simulink model "lift_stateflow"  (R2020b)
settings: Solver=VariableStepAuto  StartTime=0.0  StopTime=10.0  RelTol=1e-3
undefined symbols (not defined in the file): sigbuilder_block
libraries: simulink x2
settings Model: EnablePacing=on  PacingRate=0.100000  Creator=ADMIN  LastModifiedBy=ADMIN

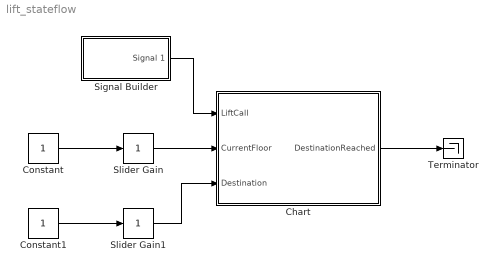
== system lift_stateflow ==
  Chart : Stateflow chart  TreatAsAtomicUnit=on
  Constant : Constant
  Constant1 : Constant
  Signal Builder : Subsystem  Tag=STV Subsys  LoadFcn=sigbuilder_block('load');  StartFcn=sigbuilder_block('start');  StopFcn=sigbuilder_block('stop');  ClipboardFcn=sigbuilder_block('clipboard');  mask(Sigbuilder block){tuvar=[0:10]}
      mask help: Simulink:masks:SigbuilderBlock_MD
      mask init:
      | if ~strcmp(get_param(bdroot(gcbh),'SimulationStatus'),'stopped') tuvar = sigbuilder_block('maskInit'); end
      settings: CopyFcn=sigbuilder_block('copy');  DeleteFcn=sigbuilder_block('delete');  ModelCloseFcn=sigbuilder_block('modelClose');  PreSaveFcn=sigbuilder_block('preSave');  PauseFcn=sigbuilder_block('pause');  ContinueFcn=sigbuilder_block('continue');  NameChangeFcn=sigbuilder_block('namechange');  OpenFcn=sigbuilder_block('open',[437.6 199.2 550.4 400 ]);  CloseFcn=sigbuilder_block('close');
      mask Display: plot(0, 0, 100, 100,[2, 2, 32, 32, 2], [68, 8, 8, 68, 68],[32, 2], [38, 38], [32, 19, 2],[53, 60, 44], [32, 17, 17, 2],[16, 16, 31, 31]);txt = getActiveGroup(gcbh);text(2, 100, txt,'verticalAlignment', 'top');
  Slider Gain : simulink/Math Operations/Slider Gain  gain=1  low=0  high=4
  Slider Gain1 : simulink/Math Operations/Slider Gain  gain=1  low=0  high=4
  Terminator : Terminator
  wires:
  Signal Builder/1(Signal 1) -> Chart/1(LiftCall)
  Slider Gain/1 -> Chart/2(CurrentFloor)
  Constant/1 -> Slider Gain/1
  Slider Gain1/1 -> Chart/3(Destination)
  Constant1/1 -> Slider Gain1/1
  Chart/1(DestinationReached) -> Terminator/1

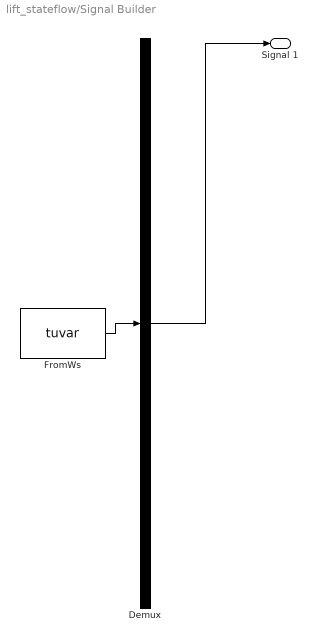
== system lift_stateflow/Signal Builder ==
  Demux : Demux  Tag=STV Demux  Outputs=1
      settings: DisplayOption=none
  FromWs : FromWorkspace  Tag=STV FromWs  VariableName=tuvar
      SigBuilderData=|
      | common.afterFinalStr = 'Extrapolate'
      | common.sampleTime = 0
      | dataSet.timeRange = [0 10]
      | dataSet.name = 'Group 1'
      | sbobj.Groups.Name = 'Group 1'
      | sbobj.Groups.Signals.Name = 'Signal 1'
      | sbobj.Groups.Signals.XData = [0 1.98 1.98 2.98 2.98 10]
      | sbobj.Groups.Signals.YData = [0 0 1 1 0 0]
  Signal 1 : Outport  Tag=STV Outport
  wires:
  Demux/1 -> Signal 1/1
  FromWs/1 -> Demux/1

== stateflow chart lift_stateflow/Chart ==
  state Stopped
    state StoppedAndWaiting
      state InitializeState
        entry:
        DestinationReached=false;
        MoveCommand=false
        Doors=false;
      state PrepareToMove
        entry:
        Doors=true;
      (default) -> InitializeState
      InitializeState -> PrepareToMove : [LiftCall]
    state StoppedAtDestination
    (default) -> StoppedAndWaiting
  state Moving
  Stopped -> Stopped [order 2] : [~LiftCall]
  (default) -> Stopped
  Moving -> StoppedAtDestination : [CurrentFloor==Destination]
  Stopped -> Moving [order 1] : [LiftCall]
  data: LiftCall input; CurrentFloor input; MoveCommand local; Doors local; Destination input; DestinationReached output
